simulink model "impedansno_upravljanje"  (R2015b)
settings: Solver=ode4  StartTime=0.0  StopTime=20  FixedStep=0.01  RelTol=1e-3
libraries: simulink x1
settings Model: Creator=Embedded Design  LastModifiedBy=Embedded Design

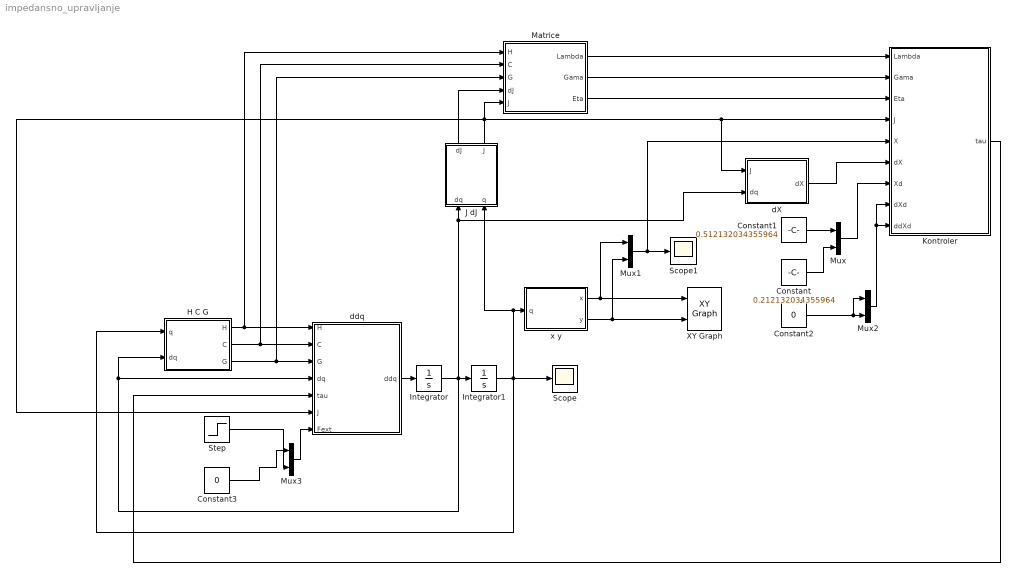
== system impedansno_upravljanje ==
  Constant : Constant  Value=0.212132034355964
  Constant1 : Constant  Value=0.512132034355964
  Constant2 : Constant  Value=0
  Constant3 : Constant  Value=0
  H C G : MATLAB Function  TreatAsAtomicUnit=on
  Integrator : Integrator  InitialCondition=[0;0]
  Integrator1 : Integrator  InitialCondition=[pi/4;pi/4]
  J dJ : MATLAB Function  TreatAsAtomicUnit=on
  Kontroler : MATLAB Function  TreatAsAtomicUnit=on
  Matrice : MATLAB Function  TreatAsAtomicUnit=on
  Mux{,1..3} (4 alike) : Mux  Inputs=2
  Scope : Scope
  Scope1 : Scope
  Step : Step  Time=2  After=-2  SampleTime=0
  XY Graph : simulink/Sinks/XY Graph  xmin=-1  xmax=1  ymin=-1  ymax=1  st=-1
  dX : MATLAB Function  TreatAsAtomicUnit=on
  ddq : MATLAB Function  TreatAsAtomicUnit=on
  x y : MATLAB Function  TreatAsAtomicUnit=on
  wires:
  H C G/1(H) -> ddq/1(H), Matrice/1(H)
  H C G/2(C) -> ddq/2(C), Matrice/2(C)
  H C G/3(G) -> ddq/3(G), Matrice/3(G)
  ddq/1(ddq) -> Integrator/1
  Integrator1/1 -> H C G/1(q), J dJ/2(q), x y/1(q), Scope/1
  Constant/1 -> Mux/2
  x y/1(x) -> XY Graph/1, Mux1/1
  x y/2(y) -> XY Graph/2, Mux1/2
  Mux1/1 -> Scope1/1, Kontroler/5(X)
  Matrice/1(Lambda) -> Kontroler/1(Lambda)
  Matrice/2(Gama) -> Kontroler/2(Gama)
  Matrice/3(Eta) -> Kontroler/3(Eta)
  J dJ/1(dJ) -> Matrice/4(dJ)
  Integrator/1 -> dX/2(dq), J dJ/1(dq), H C G/2(dq), ddq/4(dq), Integrator1/1
  Constant1/1 -> Mux/1
  Mux/1 -> Kontroler/7(Xd)
  dX/1(dX) -> Kontroler/6(dX)
  Kontroler/1(tau) -> ddq/5(tau)
  Constant2/1 -> Mux2/1, Mux2/2
  Mux2/1 -> Kontroler/8(dXd), Kontroler/9(ddXd)
  J dJ/2(J) -> ddq/6(J), Matrice/5(J), dX/1(J), Kontroler/4(J)
  Constant3/1 -> Mux3/1
  Mux3/1 -> ddq/7(Fext)
  Step/1 -> Mux3/2

== matlab function impedansno_upravljanje/ddq ==
  data: H input; ddq output; C input; G input; dq input; tau input; J input; Fext input
function ddq = fcn(H, C, G, dq, tau, J, Fext)

ddq = H^(-1)*(tau - transpose(J)*Fext - C*dq - G);

== matlab function impedansno_upravljanje/H C G ==
  data: q input; H output; dq input; C output; G output
function [H,C,G] = fcn(q,dq)

m = 4;    % [kg]
l = 0.3;  % [m]s
I = 0.03; % [kgm2]
g = 9.81; % [m/s^2]

% inertial matrix
H11 = 2*I + m*l^2*(1.5+cos(q(2)));
H12 = I + 0.5*m*l^2*(0.5+cos(q(2)));
H21 = H12;
H22 = I + 0.25*m*l^2;

H = [H11 H12;...
     H21 H22];

% velocity effects matrix
C11 = -m*l^2*sin(q(2))*dq(2);
C12 = -0.5*m*l^2*sin(q(2))*dq(2);
C21 =  0.5*m*l^2*sin(q(2))*dq(1);
C22 =  0;

C = [C11 C12;...
     C21 C22];

% gravity matrix
G11 = -1.5*m*l*g*sin(q(1))-0.5*m*l*g*sin(q(1)+q(2));
G21 = -0.5*m*l*g*sin(q(1)+q(2));

G = [G11;...
     G21];

== matlab function impedansno_upravljanje/x y ==
  data: x output; q input; y output
function [x, y] = fcn(q)

l = 0.3;  % [m]s

x = l*sin(q(1)) + l*sin(q(1) + q(2));
y = l*cos(q(1)) + l*cos(q(1) + q(2));

== matlab function impedansno_upravljanje/Kontroler ==
  data: Lambda input; Gama input; Eta input; J input; X input; dX input; Xd input; dXd input; ddXd input; tau output
function tau = fcn(Lambda, Gama, Eta, J, X, dX, Xd, dXd, ddXd)

B = [10  0; 0  10];
K = [100 0; 0 100];



tau = transpose(J)*(Lambda*ddXd + B*(dXd - dX) + K*(Xd - X) + Gama*dX +Eta);

== matlab function impedansno_upravljanje/Matrice ==
  data: H input; C input; G input; dJ input; J input; Lambda output; Gama output; Eta output
function [Lambda, Gama, Eta] = fcn(H,C,G,dJ,J)


Lambda = (transpose(J))^(-1)*H*J^(-1);
Gama = (transpose(J))^(-1)*C*J^(-1) - Lambda*dJ*J^(-1);
Eta = (transpose(J))^(-1)*G;

== matlab function impedansno_upravljanje/J dJ ==
  data: dJ output; dq input; q input; J output
function [dJ, J] = fcn(dq,q)

l = 0.3; % [m]

J = [ l*cos(q(1)) + l*cos(q(1) + q(2))   l*cos(q(1) + q(2));
     -l*sin(q(1)) - l*sin(q(1) + q(2))  -l*sin(q(1) + q(2))];
 
 dJ = [-l*sin(q(1))*dq(1) - l*sin(q(1) + q(2))*(dq(1) + dq(2)),   - l*sin(q(1) + q(2))*(dq(1) + dq(2))
       -l*cos(q(1))*dq(1) - l*cos(q(1) + q(2))*(dq(1) + dq(2)),   - l*cos(q(1) + q(2))*(dq(1) + dq(2))];

== matlab function impedansno_upravljanje/dX ==
  data: dX output; J input; dq input
function dX = fcn(J,dq)

dX = J*dq;
